simulink model "EfeitoZOH"  (R2021a)
settings: Solver=VariableStepAuto  StartTime=0.0  StopTime=10.0  RelTol=1e-3
settings Model: Creator=User  LastModifiedBy=User

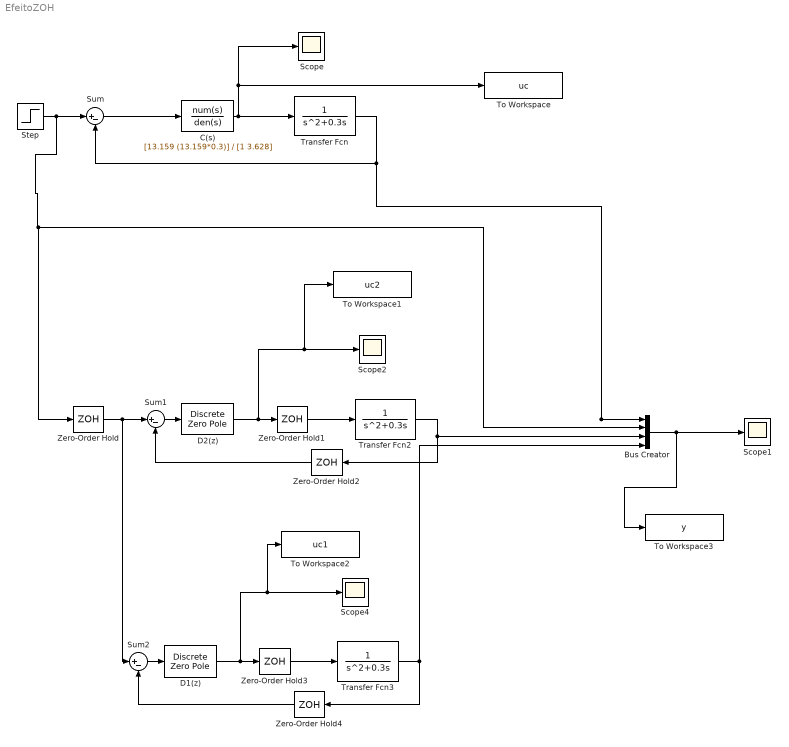
== system EfeitoZOH ==
  " C(s)" : TransferFcn  Numerator=[13.159 (13.159*0.3)]  Denominator=[1 3.628]
  Bus Creator : BusCreator  Inputs=4
  D1(z) : DiscreteZeroPole  Zeros=[0.9418]  Poles=[0.4841]  Gain=9.6414  SampleTime=-1
  D2(z) : DiscreteZeroPole  Zeros=[0.9418]  Poles=[0.3203]  Gain=9.7659  SampleTime=-1
  Scope{,1..2,4} (4 alike) : Scope
  Step : Step  SampleTime=0
  Sum : Sum  Inputs=|+-
  Sum1 : Sum  Inputs=|+-
  Sum2 : Sum  Inputs=|+-
  To Workspace : ToWorkspace  VariableName=uc  SaveFormat=Timeseries  SampleTime=-1
  To Workspace1 : ToWorkspace  VariableName=uc2  SaveFormat=Timeseries  SampleTime=-1
  To Workspace2 : ToWorkspace  VariableName=uc1  SaveFormat=Timeseries  SampleTime=-1
  To Workspace3 : ToWorkspace  VariableName=y  SaveFormat=Timeseries  SampleTime=-1
  Transfer Fcn : TransferFcn  Denominator=[1 0.3 0]
  Transfer Fcn2 : TransferFcn  Denominator=[1 0.3 0]
  Transfer Fcn3 : TransferFcn  Denominator=[1 0.3 0]
  Zero-Order Hold{,1..4} (5 alike) : ZeroOrderHold  SampleTime=-1
  wires:
  Step/1 -> Zero-Order Hold/1, Bus Creator/2, Sum/1
  Sum/1 -> " C(s)"/1
  Transfer Fcn/1 -> Bus Creator/1, Sum/2
  " C(s)"/1 -> Scope/1, To Workspace/1, Transfer Fcn/1
  Transfer Fcn2/1 -> Zero-Order Hold2/1, Bus Creator/3
  Sum1/1 -> D2(z)/1
  Zero-Order Hold2/1 -> Sum1/2
  D2(z)/1 -> To Workspace1/1, Scope2/1, Zero-Order Hold1/1
  Zero-Order Hold1/1 -> Transfer Fcn2/1
  Zero-Order Hold4/1 -> Sum2/2
  Sum2/1 -> D1(z)/1
  D1(z)/1 -> To Workspace2/1, Scope4/1, Zero-Order Hold3/1
  Zero-Order Hold3/1 -> Transfer Fcn3/1
  Zero-Order Hold/1 -> Sum2/1, Sum1/1
  Transfer Fcn3/1 -> Bus Creator/4, Zero-Order Hold4/1
  Bus Creator/1 -> To Workspace3/1, Scope1/1
